simulink model "chap6_3sim"  (Simulink 5.0)
settings: Solver=ode45  StartTime=0.0  StopTime=5  FixedStep=0.001  RelTol=1e-3
settings Model: LastModifiedBy=Administrator  ExtModeTrigMode=oneshot  ExtModeArmWhenConnect=off  LimitDataPoints=off  BooleanDataType=off

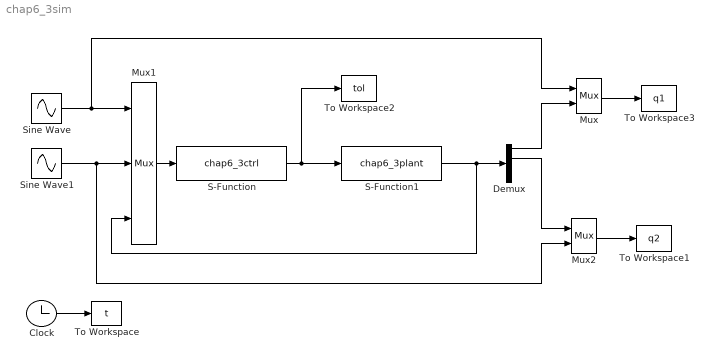
== system chap6_3sim ==
  Clock : Clock
  Demux : Demux
  Mux : Mux  Inputs=2
  Mux1 : Mux  Inputs=3
  Mux2 : Mux  Inputs=2
  S-Function : S-Function  FunctionName=chap6_3ctrl
  S-Function1 : S-Function  FunctionName=chap6_3plant
  Sine Wave : Sin  Frequency=2*pi  SampleTime=0
  Sine Wave1 : Sin  Frequency=2*pi  SampleTime=0
  To Workspace : ToWorkspace  VariableName=t  SampleTime=-1  SaveFormat=Array
  To Workspace1 : ToWorkspace  VariableName=q2  SampleTime=-1  SaveFormat=Array
  To Workspace2 : ToWorkspace  VariableName=tol  SampleTime=-1  SaveFormat=Array
  To Workspace3 : ToWorkspace  VariableName=q1  SampleTime=-1  SaveFormat=Array
  wires:
  Mux1/1 -> S-Function/1
  S-Function/1 -> S-Function1/1, To Workspace2/1
  Sine Wave/1 -> Mux/1, Mux1/1
  Mux/1 -> To Workspace3/1
  Demux/1 -> Mux/2
  S-Function1/1 -> Demux/1, Mux1/3
  Clock/1 -> To Workspace/1
  Sine Wave1/1 -> Mux1/2, Mux2/2
  Mux2/1 -> To Workspace1/1
  Demux/2 -> Mux2/1
